simulink model "cartpole"  (R2022b)
settings: Solver=FixedStepAuto  StartTime=0.0  StopTime=10.0  FixedStep=0.02  RelTol=1e-3
model workspace (MAT data in the model file):
  a_max = 30
  a_min = -30
  adva_max = 1
  adva_min = -1
  g = 9.8
  l_cg = 0.5
  m_cart = 1
  m_pendulum = 0.1
  x_ini = Simulink.Parameter
  x_ini.Value = [0 0 0 0]
  x_ini.DataType = 'auto'
  x_ini.Complexity = 'real'
  x_ini.Dimensions = [1 4]
  x_max = [4.8 9999 0.4 9999]
  x_min = [-4.8 -9999 -0.4 -9999]
libraries: simulink x1
settings Model: TunableVars=a_max,a_min,adva_max,adva_min,x_ini,x_max,x_min  TunableVarsStorageClass=Auto,Auto,Auto,Auto,Auto,Auto,Auto  TunableVarsTypeQualifier=,,,,,,  ParameterArgumentNames=x_ini  Creator=hjzsj  LastModifiedBy=Yuxuan
settings ConfigSet: Description=Config for code generation python binding.
settings SolverCC: AlgebraicLoopSolver=TrustRegion
settings OptimizationCC: DefaultParameterBehavior=Inlined  UseDivisionForNetSlopeComputation=on  UseFloatMulNetSlope=on  StrengthReduction=on  PassReuseOutputArgsAs=Individual arguments  ZeroExternalMemoryAtStartup=off  ZeroInternalMemoryAtStartup=off  NoFixptDivByZeroProtection=on  EfficientFloat2IntCast=on  OptimizeBlockOrder=speed  OptimizationPriority=Speed  OptimizationCustomize=off  MultiThreadedLoops=on  EfficientTunableParamExpr=on
settings DebuggingCC: ParameterTunabilityLossMsg=error  UnconnectedInputMsg=warning  UnconnectedOutputMsg=warning  UnconnectedLineMsg=warning  SFMachineParentedDataDiag=warning  ArithmeticOperatorsInVariantConditions=warning
settings HardwareCC: ProdLongLongMode=on  TargetPreprocMaxBitsSint=64  TargetPreprocMaxBitsUint=64
settings ModelReferenceCC: EnableRefExpFcnMdlSchedulingChecks=on
settings SFSimCC: MATLABDynamicMemAlloc=off  CustomCodeUndefinedFunction=UseInterfaceOnly  SimTargetLang=C++
settings RTWCC: Description=Embedded Coder  SystemTargetFile=ert.tlc  GenCodeOnly=on  TemplateMakefile=ert_default_tmf  PostCodeGenCommand=slxpy.postprocess(modelName,buildInfo)  RetainRTWFile=on  PortableWordSizes=on  TargetLang=C++
settings CodeAppCC: ForceParamTrailComments=on  CommentStyle=Multi-line  IgnoreCustomStorageClasses=off  MaxIdLength=64  OperatorAnnotations=on  SimulinkDataObjDesc=on  SFDataObjDesc=on  MATLABFcnDesc=on  MangleLength=4  InsertBlockDesc=on  StateflowObjectComments=on  MATLABSourceComments=on
settings ERTTargetCC: TargetLangStandard=C++11 (ISO)  SupportAbsoluteTime=off  CodeInterfacePackaging=C++ class  SupportNonFinite=off  SupportComplex=off  SupportContinuousTime=on  InlinedParameterPlacement=NonHierarchical  RootIOFormat=Structure reference  ERTCustomFileTemplate=example_file_process.tlc

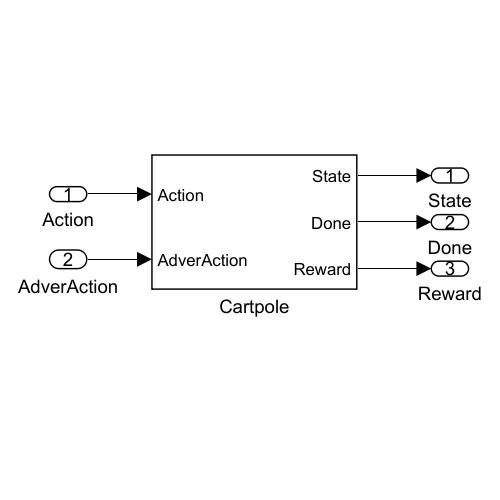
[thumbnail: Simulink's stored preview of the top-level diagram]
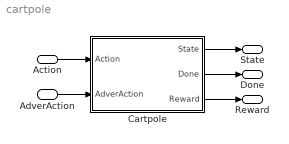
== system cartpole ==
  Action : Inport
  AdverAction : Inport  Port=2
  "Cartpole " : Subsystem
  State : Outport
  Done : Outport  Port=2
  Reward : Outport  Port=3
  wires:
  "Cartpole "/1(State) -> State/1
  "Cartpole "/2(Done) -> Done/1
  Action/1 -> "Cartpole "/1(Action)
  "Cartpole "/3(Reward) -> Reward/1
  AdverAction/1 -> "Cartpole "/2(AdverAction)

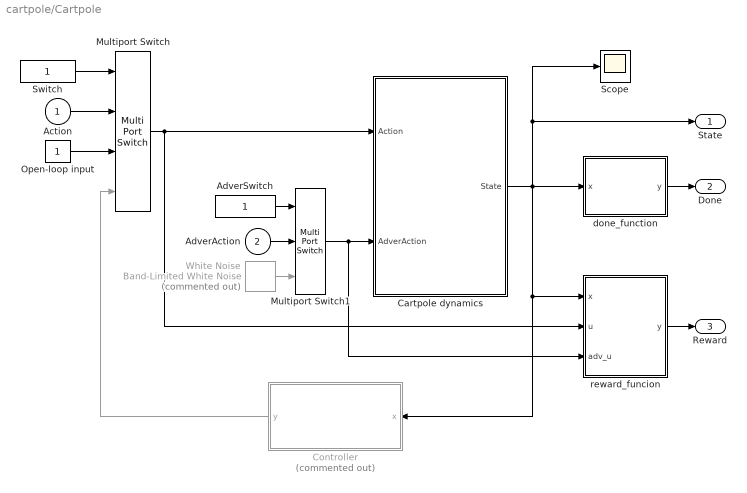
== system cartpole/Cartpole  ==
  Action : Inport
  AdverAction : Inport  Port=2
  AdverSwitch : Constant
  "Cartpole dynamics " : Subsystem
  Controller : MATLAB Function  Commented=on  TreatAsAtomicUnit=on
  Multiport Switch : MultiPortSwitch  SaturateOnIntegerOverflow=off  InputSameDT=off
  Multiport Switch1 : MultiPortSwitch  Inputs=2  SaturateOnIntegerOverflow=off  InputSameDT=off
  Open-loop input : Constant
  Scope : Scope
  Switch : Constant
  White Noise : simulink/Sources/Band-Limited White Noise  Commented=on  Cov=[0.5]  Ts=0.02  seed=[23341]
  "done_function " : MATLAB Function  TreatAsAtomicUnit=on
  "reward_funcion " : MATLAB Function  TreatAsAtomicUnit=on
  State : Outport
  Done : Outport  Port=2
  Reward : Outport  Port=3
  wires:
  "done_function "/1(y) -> Done/1
  Multiport Switch/1 -> "Cartpole dynamics "/1("Action "), "reward_funcion "/2(u)
  "Cartpole dynamics "/1(State) -> Controller/1(x), "reward_funcion "/1(x), "done_function "/1(x), State/1, Scope/1
  "reward_funcion "/1(y) -> Reward/1
  Action/1 -> Multiport Switch/2
  Switch/1 -> Multiport Switch/1
  Open-loop input/1 -> Multiport Switch/3
  Controller/1(y) -> Multiport Switch/4
  AdverSwitch/1 -> Multiport Switch1/1
  Multiport Switch1/1 -> "reward_funcion "/3(adv_u), "Cartpole dynamics "/2(AdverAction)
  AdverAction/1 -> Multiport Switch1/2
  White Noise/1 -> Multiport Switch1/3

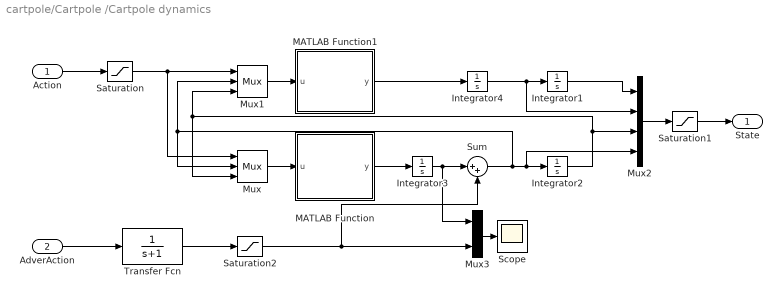
== system cartpole/Cartpole /Cartpole dynamics  ==
  "Action " : Inport
  AdverAction : Inport  Port=2
  Integrator1 : Integrator  InitialCondition=x_ini(1)
  Integrator2 : Integrator  InitialCondition=x_ini(3)
  Integrator3 : Integrator  InitialCondition=x_ini(4)
  Integrator4 : Integrator  InitialCondition=x_ini(2)
  MATLAB Function : MATLAB Function  TreatAsAtomicUnit=on
  MATLAB Function1 : MATLAB Function  TreatAsAtomicUnit=on
  Mux : Mux  Inputs=3
  Mux1 : Mux  Inputs=3
  Mux2 : Mux
  Mux3 : Mux  Inputs=2
  Saturation : Saturate  UpperLimit=a_max  LowerLimit=a_min
  Saturation1 : Saturate  UpperLimit=x_max  LowerLimit=x_min
  Saturation2 : Saturate  UpperLimit=adva_max  LowerLimit=adva_min
  Scope : Scope
  Sum : Sum  Inputs=|++
  Transfer Fcn : TransferFcn  Denominator=[1 1]
  State : Outport  VectorParamsAs1DForOutWhenUnconnected=off
  wires:
  MATLAB Function1/1(y) -> Integrator4/1
  Mux1/1 -> MATLAB Function1/1(u)
  Integrator1/1 -> Mux2/1
  Integrator4/1 -> Mux2/2, Integrator1/1
  Integrator2/1 -> Mux1/3, Mux/3, Mux2/3
  Mux/1 -> MATLAB Function/1(u)
  Sum/1 -> Mux2/4, Integrator2/1, Mux1/2, Mux/2
  Saturation/1 -> Mux1/1, Mux/1
  Mux2/1 -> Saturation1/1
  "Action "/1 -> Saturation/1
  Saturation1/1 -> State/1
  AdverAction/1 -> Transfer Fcn/1
  MATLAB Function/1(y) -> Integrator3/1
  Saturation2/1 -> Sum/2, Mux3/2
  Mux3/1 -> Scope/1
  Integrator3/1 -> Mux3/1, Sum/1
  Transfer Fcn/1 -> Saturation2/1

== matlab function cartpole/Cartpole /reward_funcion  ==
  data: x input size=4; y output; u input size=1; adv_u input
function y = fcn(x, u, adv_u)
done = (abs(x(1)) > 2.4)||(abs(x(3)) > 0.2094);
y = 1 - double(done);

== matlab function cartpole/Cartpole /Controller ==
  data: x input size=4; y output
function y = fcn(x)
done = (abs(x(1)) > 2.4)||(abs(x(3)) > 0.2094);
y = done;

== matlab function cartpole/Cartpole /Cartpole dynamics /MATLAB Function ==
  data: u input size=3; y output; m_pendulum parameter; m_cart parameter; g parameter; l_cg parameter
function y = fcn(u, m_pendulum, m_cart, g, l_cg)
y = (-u(1)*cos(u(3))/m_pendulum + (m_cart+m_pendulum)*g*sin(u(3))/m_pendulum - l_cg*power(u(2),2)*sin(u(3))*cos(u(3)))/(l_cg*(m_cart/m_pendulum + power(sin(u(3)),2)));

== matlab function cartpole/Cartpole /Cartpole dynamics /MATLAB Function1 ==
  data: u input size=3; y output; m_pendulum parameter; m_cart parameter; g parameter; l_cg parameter
function y = fcn(u, m_pendulum, m_cart, g, l_cg)
y = (u(1)/m_pendulum - g*sin(u(3))*cos(u(3)) + l_cg*power(u(2),2)*sin(u(3)))/(m_cart/m_pendulum + power(sin(u(3)),2));

== matlab function cartpole/Cartpole /done_function  ==
  data: x input size=4; y output
function y = fcn(x)
done = (abs(x(1)) > 2.4)||(abs(x(3)) > 0.2094);
y = done;
